simulink model "Optimized_PWM"  (R2019a)
settings: Solver=ode45  StartTime=0.0  StopTime=0.2  MaxStep=1e-4  RelTol=1e-3
values from neighbouring files (symbols this model uses):
  alpha_op_1 = alphas1_sorted(1)    [inputs.m]    (also in solve_harmonics_optimized.m = alphas(1))
  alpha_op_2 = alphas1_sorted(2)    [inputs.m]    (also in solve_harmonics_optimized.m = alphas(2))
  alpha_op_3 = alphas1_sorted(3)    [inputs.m]    (also in solve_harmonics_optimized.m = alphas(3))
  f = 50    [inputs.m]
  L = 33e-3    (= 0.033)    [inputs.m]
  R = 33    [inputs.m]
  Vdc = 100    [inputs.m]
libraries: powerlib x10
settings Model: Creator=omar_  LastModifiedBy=omar_
settings DataIOCC: ReturnWorkspaceOutputs=off

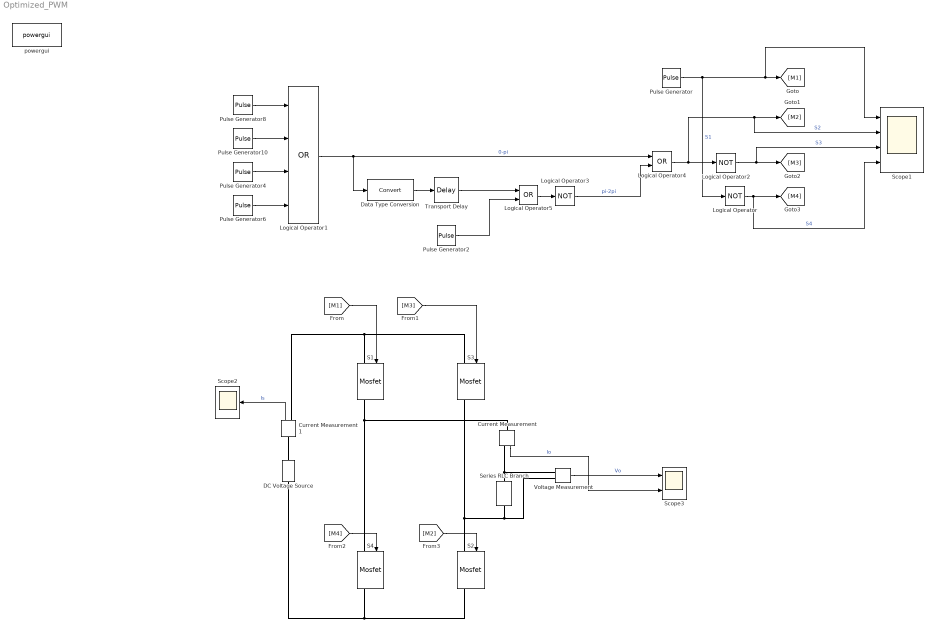
== system Optimized_PWM ==
  Current Measurement : powerlib/Measurements/Current Measurement  PhasorSimulation=off  OutputType=Magnitude  PSBequivalent=0
      settings: SourceProductName=Simscape Electrical
  Current Measurement1 : powerlib/Measurements/Current Measurement  PhasorSimulation=off  OutputType=Magnitude  PSBequivalent=0
      settings: SourceProductName=Simscape Electrical
  DC Voltage Source : powerlib/Electrical Sources/DC Voltage Source  Amplitude=Vdc  Measurements=None
      settings: SourceProductName=Simscape Electrical
  Data Type Conversion : DataTypeConversion
  Logical Operator : Logic  Operator=NOT  AllPortsSameDT=off  OutDataTypeStr=boolean
  Logical Operator1 : Logic  Operator=OR  Inputs=4  AllPortsSameDT=off  OutDataTypeStr=boolean
  Logical Operator2 : Logic  Operator=NOT  AllPortsSameDT=off  OutDataTypeStr=boolean
  Logical Operator3 : Logic  Operator=NOT  AllPortsSameDT=off  OutDataTypeStr=boolean
  Logical Operator4 : Logic  Operator=OR  AllPortsSameDT=off  OutDataTypeStr=boolean
  Logical Operator5 : Logic  Operator=OR  AllPortsSameDT=off  OutDataTypeStr=boolean
  Pulse Generator : DiscretePulseGenerator  PulseType=Time based  Period=1/f  PulseWidth=50
  Pulse Generator10 : DiscretePulseGenerator  PulseType=Time based  Period=1/f  PulseWidth=((90-alpha_op_3)/360)*100  PhaseDelay=((alpha_op_3)/180)/100
  Pulse Generator2 : DiscretePulseGenerator  PulseType=Time based  Period=1/f  PulseWidth=50
  Pulse Generator4 : DiscretePulseGenerator  PulseType=Time based  Period=1/f  PulseWidth=((90-alpha_op_3)/360)*100  PhaseDelay=1/200
  Pulse Generator6 : DiscretePulseGenerator  PulseType=Time based  Period=1/f  PulseWidth=((alpha_op_2-alpha_op_1)/360)*100  PhaseDelay=((180-alpha_op_2)/180)/100
  Pulse Generator8 : DiscretePulseGenerator  PulseType=Time based  Period=1/f  PulseWidth=((alpha_op_2-alpha_op_1)/360)*100  PhaseDelay=((alpha_op_1)/180)/100
  S{1..4} (4 alike) : powerlib/Power Electronics/Mosfet  Ron=0.1  Lon=0  Rd=0.01  Vfd=0  IC=0  Rs=1e5  Cs=inf  Measurements=on
      settings: SourceProductName=Simscape Electrical
  Scope1 : Scope  NumInputPorts=4
  Scope2 : Scope
  Scope3 : Scope  NumInputPorts=2
  Series RLC Branch : powerlib/Elements/Series RLC Branch  LConnTagsString=__new0  RConnTagsString=__new0  BranchType=RL  Resistance=R  Inductance=L  SetiL0=off  InitialCurrent=0  Capacitance=1e-6  Setx0=off  InitialVoltage=0  Measurements=None
      settings: SourceProductName=Simscape Electrical
  Transport Delay : TransportDelay  DelayTime=0.01  InitialOutput=0.01
  Voltage Measurement : powerlib/Measurements/Voltage Measurement  PhasorSimulation=off  OutputType=Magnitude  PSBequivalent=0
      settings: SourceProductName=Simscape Electrical
  powergui : powerlib/powergui  Priority=1  SimulationMode=Continuous  SampleTime=50e-8  frequency=60  Iterations=50  frequencyindice=0  Pbase=100e6  ErrMax=1e-4  UnitsV=kV  UnitsW=MW  buscounter=0  FunctionMessages=off  echomessages=off  EnableUseOfTLC=off  CurrentSourceSwitches=off  DisableSnubberDevices=off  DisableRonSwitches=off  DisableVfSwitches=off  DisplayEquations=off  AutomaticDiscreteSolvers=off  SolverType=Tustin/Backward Euler (TBE)  Interpol=off  ExternalGateDelay=off  methode=off  Ts=100  x0status=blocks  SPID=on  SwTol=0  HookPort=off  NonlinearTolerance=0  nMaxIteration=15  ContinueOnMaxIteration=off  RestoreLinks=warning  ResistiveCurrentMeasurement=off  Frange=[0:2:500]  Ylog=off  Xlog=on  ShowGrid=off  save=off  variable=ZData  structure=Outputs  ZoomFFT=off  StartTime=0.08  cycles=3  DisplayStyle=2  fundamental=50  FreqAxis=off  MaxFrequency=1000  frequencyindicesteady=1  RmsSteady=1  display=off
      settings: SourceProductName=Simscape Electrical
  wires:
  Voltage Measurement/1 -> Scope3/1  "Vo"
  [M1] -> S1/1
  Current Measurement/1 -> Scope3/2  "Io"
  Current Measurement1/1 -> Scope2/1  "Is"
  [M2] -> S2/1
  [M4] -> S4/1
  [M3] -> S3/1
  Logical Operator/1 -> Scope1/4, [M4]  "S4"
  Pulse Generator/1 -> Logical Operator/1, Scope1/1, [M1]  "S1"
  Logical Operator2/1 -> [M3], Scope1/3  "S3"
  Logical Operator4/1 -> Scope1/2, [M2], Logical Operator2/1  "S2"
  Logical Operator1/1 -> Data Type Conversion/1, Logical Operator4/1  "0-pi"
  Data Type Conversion/1 -> Transport Delay/1
  Pulse Generator2/1 -> Logical Operator5/2
  Transport Delay/1 -> Logical Operator5/1
  Logical Operator5/1 -> Logical Operator3/1
  Logical Operator3/1 -> Logical Operator4/2  "pi-2pi"
  Pulse Generator6/1 -> Logical Operator1/4
  Pulse Generator4/1 -> Logical Operator1/3
  Pulse Generator10/1 -> Logical Operator1/2
  Pulse Generator8/1 -> Logical Operator1/1
  connections:
  Current Measurement/LConn1 -- S1/RConn1 -- S4/LConn1
  Current Measurement1/RConn1 -- S3/LConn1 -- S1/LConn1
  S4/RConn1 -- S2/RConn1 -- DC Voltage Source/LConn1
  Voltage Measurement/LConn2 -- S2/LConn1 -- S3/RConn1 -- Series RLC Branch/RConn1
  Voltage Measurement/LConn1 -- Series RLC Branch/LConn1 -- Current Measurement/RConn1
  Current Measurement1/LConn1 -- DC Voltage Source/RConn1
